simulink model "Subsystem"  (R2020a)
settings: Solver=VariableStepAuto  StartTime=0.0  StopTime=10.0  RelTol=1e-3
settings Model: Creator=DELL  LastModifiedBy=DELL
settings DataIOCC: SaveOutput=off  SaveTime=off

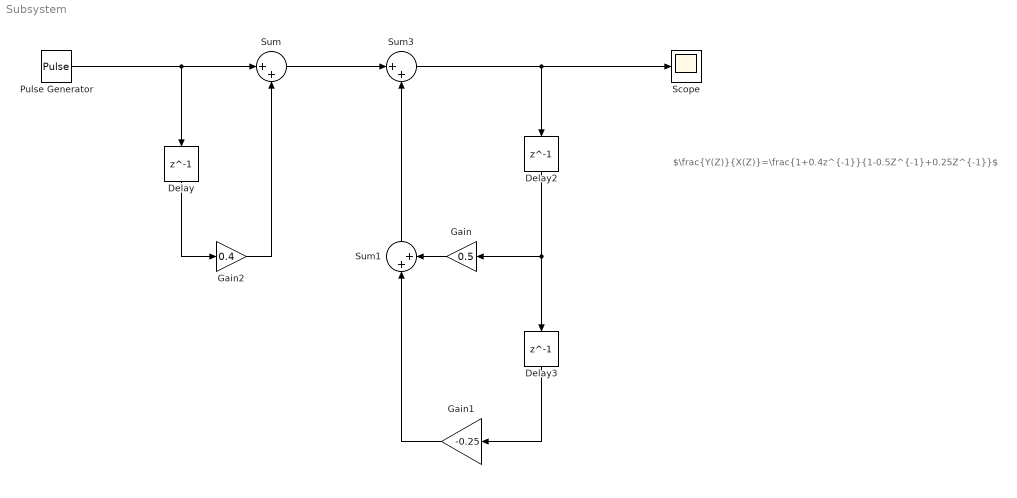
== system Subsystem ==
  note: $\frac{Y(Z)}{X(Z)}=\frac{1+0.4z^{-1}}{1-0.5Z^{-1}+0.25Z^{-1}}$
  Delay : Delay  DelayLength=1
  Delay2 : Delay  DelayLength=1
  Delay3 : Delay  DelayLength=1
  Gain : Gain  Gain=0.5
  Gain1 : Gain  Gain=-0.25
  Gain2 : Gain  Gain=0.4
  Pulse Generator : DiscretePulseGenerator  PulseType=Time based  Period=10  PulseWidth=5
  Scope : Scope
  Sum : Sum  Inputs=|++
  Sum1 : Sum  Inputs=|++
  Sum3 : Sum  Inputs=|++
  wires:
  Sum3/1 -> Delay2/1, Scope/1
  Pulse Generator/1 -> Delay/1, Sum/1
  Gain/1 -> Sum1/2
  Sum1/1 -> Sum3/2
  Delay2/1 -> Gain/1, Delay3/1
  Gain1/1 -> Sum1/1
  Gain2/1 -> Sum/2
  Delay3/1 -> Gain1/1
  Sum/1 -> Sum3/1
  Delay/1 -> Gain2/1
